simulink model "DroneControl_copy"  (R2023a)
settings: Solver=VariableStepAuto  StartTime=0.0  StopTime=Tfinal  RelTol=1e-3
values from neighbouring files (symbols this model uses):
  body_rate_0 = [0 0 ... (first row only)    [XYZsignal_copy.m]
  Euler_0 = [0 0 ... (first row only)    [XYZsignal_copy.m]
  g = [0;0;-9.8]    [XYZsignal_copy.m]
  I = [[0.1,0,0];[0,0.1,0];[0,0,0.08]]    [XYZsignal_copy.m]
  m = 0.2    [XYZsignal_copy.m]    (also in animation_copy.m = T_V1toI*T_V2toV1*T_BtoV2)
  surround_rate = 0    [XYZsignal_copy.m]
  ts = 0.01    [XYZsignal_copy.m]
  Xcmd1 = timeseries(sigX1(2:end,:),sigX1(1,:))    [XYZsignal_copy.m]
  Xcmd2 = timeseries(sigX2(2:end,:),sigX2(1,:))    [XYZsignal_copy.m]
  XYZ_0 = [0.1 10.1 ... (first row only)    [XYZsignal_copy.m]
  Ycmd1 = timeseries(sigY1(2:end,:),sigY1(1,:))    [XYZsignal_copy.m]
  Ycmd2 = timeseries(sigY2(2:end,:),sigY2(1,:))    [XYZsignal_copy.m]
libraries: slpidlib x36, vrlib x4, simulink_extras x2
(part 1 of 5)
settings Model: NumberOfSteps=10  Creator=blaze8871  LastModifiedBy=sujay
settings SolverCC: AlgebraicLoopSolver=TrustRegion
settings DataIOCC: SaveTime=off
settings DebuggingCC: UnconnectedInputMsg=warning  UnconnectedOutputMsg=warning  UnconnectedLineMsg=warning
settings ModelReferenceCC: EnableRefExpFcnMdlSchedulingChecks=on

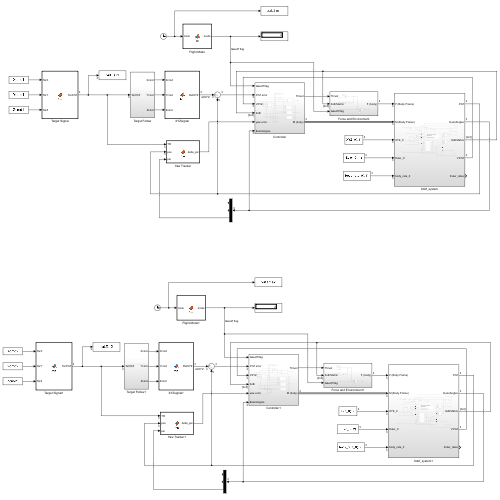
[thumbnail: Simulink's stored preview of the top-level diagram]
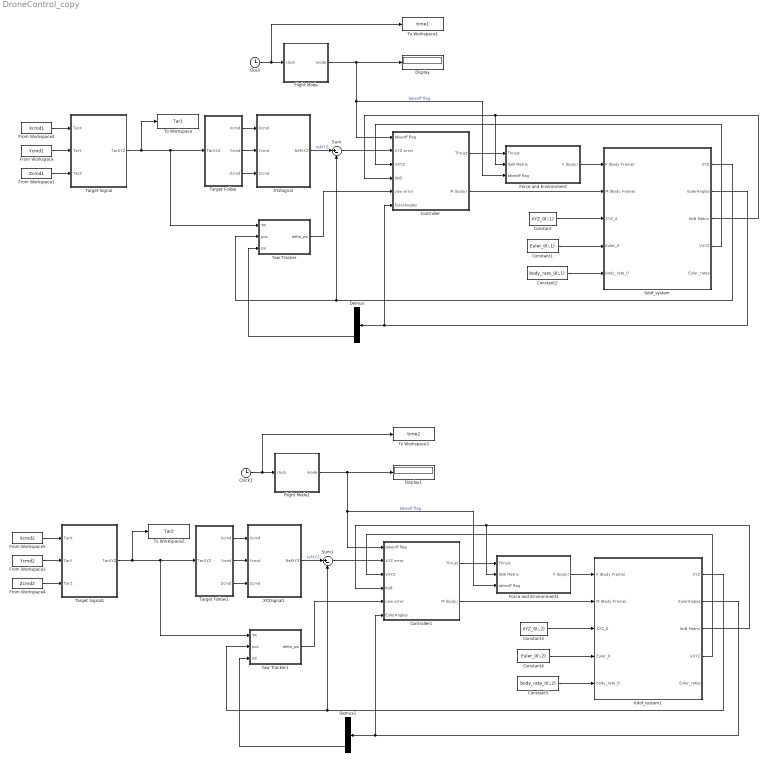
== system DroneControl_copy ==
  6dof_system : Subsystem
  6dof_system1 : Subsystem
  Clock : Clock
  Clock1 : Clock
  Constant : Constant  Value=XYZ_0(:,1)  SampleTime=0.01
  Constant1 : Constant  Value=Euler_0(:,1)  SampleTime=0.01
  Constant2 : Constant  Value=body_rate_0(:,1)  SampleTime=0.01
  Constant3 : Constant  Value=XYZ_0(:,2)  SampleTime=0.01
  Constant4 : Constant  Value=Euler_0(:,2)  SampleTime=0.01
  Constant5 : Constant  Value=body_rate_0(:,2)  SampleTime=0.01
  Controller : Subsystem
  Controller1 : Subsystem
  Demux : Demux  Outputs=3
  Demux1 : Demux  Outputs=3
  Display : Display
  Display1 : Display
  Flight Mode : MATLAB Function  TreatAsAtomicUnit=on
  Flight Mode1 : MATLAB Function  TreatAsAtomicUnit=on
  Force and Environment : Subsystem
  Force and Environment1 : Subsystem
  From Workspace : FromWorkspace  VariableName=Ycmd1  SampleTime=ts
  From Workspace1 : FromWorkspace  VariableName=Zcmd1  SampleTime=ts
  From Workspace2 : FromWorkspace  VariableName=Xcmd1  SampleTime=ts
  From Workspace3 : FromWorkspace  VariableName=Ycmd2  SampleTime=ts
  From Workspace4 : FromWorkspace  VariableName=Zcmd2  SampleTime=ts
  From Workspace5 : FromWorkspace  VariableName=Xcmd2  SampleTime=ts
  Sum : Sum  Inputs=|+-
  Sum1 : Sum  Inputs=|+-
  Target Follow : Subsystem
  Target Follow1 : Subsystem
  Target Signal : MATLAB Function  TreatAsAtomicUnit=on
  Target Signal1 : MATLAB Function  TreatAsAtomicUnit=on
  To Workspace : ToWorkspace  VariableName=Tar1  SampleTime=ts
  To Workspace1 : ToWorkspace  VariableName=time1  SampleTime=ts
  To Workspace2 : ToWorkspace  VariableName=Tar2  SampleTime=ts
  To Workspace3 : ToWorkspace  VariableName=time2  SampleTime=ts
  XYZsignal : MATLAB Function  TreatAsAtomicUnit=on
  XYZsignal1 : MATLAB Function  TreatAsAtomicUnit=on
  Yaw Tracker : MATLAB Function  TreatAsAtomicUnit=on
  Yaw Tracker1 : MATLAB Function  TreatAsAtomicUnit=on
  wires:
  Constant/1 -> 6dof_system/3(XYZ_0)
  Constant1/1 -> 6dof_system/4(Euler_0)
  Constant2/1 -> 6dof_system/5(body_rate_0)
  6dof_system/3(ItoB Matrix) -> Force and Environment/2(ItoB Matrix), Controller/4(ItoB)
  XYZsignal/1(RefXYZ) -> Sum/1  "refXYZ"
  6dof_system/1(XYZ) -> Sum/2, Yaw Tracker/2(pos)
  Clock/1 -> To Workspace1/1, Flight Mode/1(clock)
  Flight Mode/1(mode) -> Controller/1(takeoff flag), Force and Environment/3(takeoff flag), Display/1  "takeoff flag"
  Force and Environment/1(F (body)) -> 6dof_system/1(F (Body Frame))
  6dof_system/2(EulerAngles) -> Controller/6(EulerAngles), Demux/1
  Sum/1 -> Controller/2(XYZ error)
  6dof_system/4(VXYZ) -> Controller/3(VXYZ)
  Controller/2(M (body)) -> 6dof_system/2(M (Body Frame))
  Controller/1(Thrust) -> Force and Environment/1(Thrust)
  Demux/3 -> Yaw Tracker/3(psi)
  Yaw Tracker/1(delta_psi) -> Controller/5(yaw error)
  Target Signal/1(TarXYZ) -> To Workspace/1, Target Follow/1(TarXYZ), Yaw Tracker/1(TR)
  From Workspace2/1 -> Target Signal/1(TarX)
  From Workspace/1 -> Target Signal/2(TarY)
  From Workspace1/1 -> Target Signal/3(TarZ)
  Target Follow/1(Xcmd) -> XYZsignal/1(Xcmd)
  Target Follow/2(Ycmd) -> XYZsignal/2(Ycmd)
  Target Follow/3(Zcmd) -> XYZsignal/3(Zcmd)
  Controller1/2(M (body)) -> 6dof_system1/2(M (Body Frame))
  Demux1/3 -> Yaw Tracker1/3(psi)
  Yaw Tracker1/1(delta_psi) -> Controller1/5(yaw error)
  Controller1/1(Thrust) -> Force and Environment1/1(Thrust)
  From Workspace3/1 -> Target Signal1/2(TarY)
  Force and Environment1/1(F (body)) -> 6dof_system1/1(F (Body Frame))
  Target Signal1/1(TarXYZ) -> To Workspace2/1, Target Follow1/1(TarXYZ), Yaw Tracker1/1(TR)
  Target Follow1/3(Zcmd) -> XYZsignal1/3(Zcmd)
  Target Follow1/1(Xcmd) -> XYZsignal1/1(Xcmd)
  From Workspace4/1 -> Target Signal1/3(TarZ)
  From Workspace5/1 -> Target Signal1/1(TarX)
  Constant3/1 -> 6dof_system1/3(XYZ_0)
  6dof_system1/4(VXYZ) -> Controller1/3(VXYZ)
  6dof_system1/2(EulerAngles) -> Controller1/6(EulerAngles), Demux1/1
  XYZsignal1/1(RefXYZ) -> Sum1/1  "refXYZ"
  6dof_system1/3(ItoB Matrix) -> Force and Environment1/2(ItoB Matrix), Controller1/4(ItoB)
  Flight Mode1/1(mode) -> Controller1/1(takeoff flag), Force and Environment1/3(takeoff flag), Display1/1  "takeoff flag"
  Sum1/1 -> Controller1/2(XYZ error)
  Constant4/1 -> 6dof_system1/4(Euler_0)
  Constant5/1 -> 6dof_system1/5(body_rate_0)
  Clock1/1 -> To Workspace3/1, Flight Mode1/1(clock)
  Target Follow1/2(Ycmd) -> XYZsignal1/2(Ycmd)
  6dof_system1/1(XYZ) -> Sum1/2, Yaw Tracker1/2(pos)

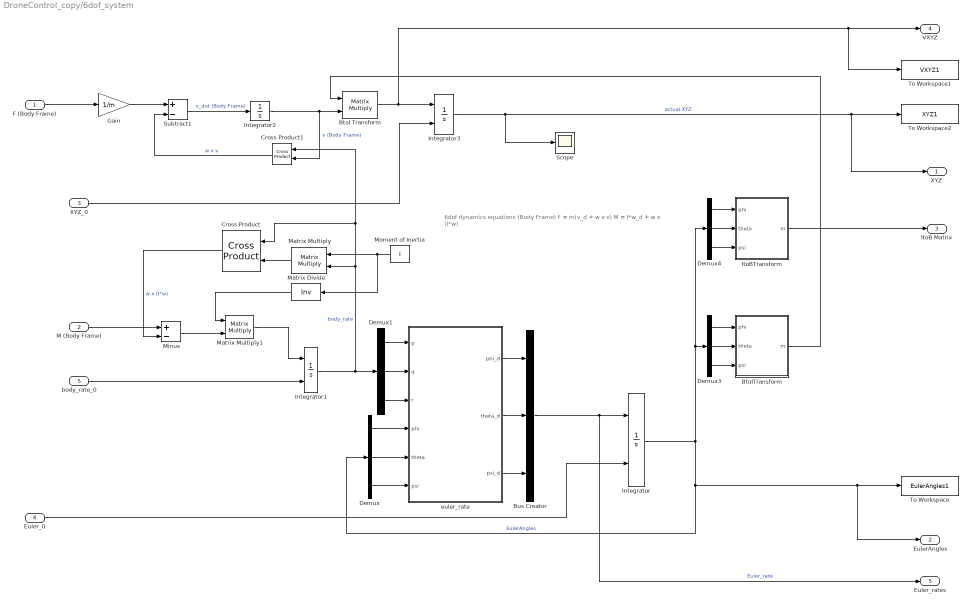
== system DroneControl_copy/6dof_system ==
  note: 6dof dynamics equations
      | (Body Frame)
      |
      | F = m(v_d + w x v)
      | M = I*w_d + w x (I*w)
  F (Body Frame) : Inport
  M (Body Frame) : Inport  Port=2
  XYZ_0 : Inport  Port=3
  Euler_0 : Inport  Port=4
  body_rate_0 : Inport  Port=5
  BtoI Transform : Product  Multiplication=Matrix(*)
  BtoITransform : MATLAB Function  TreatAsAtomicUnit=on
  Bus Creator : BusCreator  Inputs=3
  Cross Product : vrlib/Utilities/Cross Product
  Cross Product1 : vrlib/Utilities/Cross Product
  Demux{,1,3..4} (4 alike) : Demux  Outputs=3
  Gain : Gain  Gain=1/m
  Integrator : Integrator  InitialConditionSource=external  ContinuousStateAttributes='EulerAngle'
  Integrator1 : Integrator  InitialConditionSource=external  ContinuousStateAttributes='EulerAngle'
  Integrator2 : Integrator
  Integrator3 : Integrator  InitialConditionSource=external
  ItoBTransform : MATLAB Function  TreatAsAtomicUnit=on
  Matrix Divide : Product  Inputs=/  Multiplication=Matrix(*)
  Matrix Multiply : Product  Multiplication=Matrix(*)
  Matrix Multiply1 : Product  Multiplication=Matrix(*)
  Minus : Sum  Inputs=+-
  Moment of Inertia : Constant  Value=I
  Scope : Scope
  Subtract1 : Sum  Inputs=+-
  To Workspace : ToWorkspace  VariableName=EulerAngles1  SampleTime=ts
  To Workspace1 : ToWorkspace  VariableName=VXYZ1  SampleTime=ts
  To Workspace2 : ToWorkspace  VariableName=XYZ1  SampleTime=ts
  euler_rate : MATLAB Function  TreatAsAtomicUnit=on
  XYZ : Outport
  EulerAngles : Outport  Port=2
  ItoB Matrix : Outport  Port=3
  VXYZ : Outport  Port=4
  Euler_rates : Outport  Port=5
  wires:
  F (Body Frame)/1 -> Gain/1
  Demux4/2 -> ItoBTransform/2(theta)
  euler_rate/1(phi_d) -> Bus Creator/1
  BtoITransform/1(m) -> BtoI Transform/1
  Bus Creator/1 -> Euler_rates/1, Integrator/1  "Euler_rate"
  Matrix Multiply/1 -> Cross Product/2
  Moment of Inertia/1 -> Matrix Divide/1, Matrix Multiply/1
  Demux3/2 -> BtoITransform/2(theta)
  Demux/2 -> euler_rate/5(theta)
  Demux4/1 -> ItoBTransform/1(phi)
  Subtract1/1 -> Integrator2/1  "v_dot (Body Frame)"
  Cross Product1/1 -> Subtract1/2  "w x v"
  Demux1/1 -> euler_rate/1(p)
  Demux/3 -> euler_rate/6(psi)
  euler_rate/2(theta_d) -> Bus Creator/2
  Euler_0/1 -> Integrator/2
  Integrator3/1 -> XYZ/1, To Workspace2/1, Scope/1  "actual XYZ"
  Cross Product/1 -> Minus/2  "w x (I*w)"
  M (Body Frame)/1 -> Minus/1
  body_rate_0/1 -> Integrator1/2
  Demux3/3 -> BtoITransform/3(psi)
  euler_rate/3(psi_d) -> Bus Creator/3
  Demux4/3 -> ItoBTransform/3(psi)
  Gain/1 -> Subtract1/1
  Demux3/1 -> BtoITransform/1(phi)
  Demux1/3 -> euler_rate/3(r)
  XYZ_0/1 -> Integrator3/2
  Integrator/1 -> EulerAngles/1, To Workspace/1, Demux/1, Demux4/1, Demux3/1  "EulerAngles"
  Demux/1 -> euler_rate/4(phi)
  Integrator2/1 -> BtoI Transform/2, Cross Product1/2  "v (Body Frame)"
  Integrator1/1 -> Cross Product1/1, Cross Product/1, Matrix Multiply/2, Demux1/1  "body_rate"
  Demux1/2 -> euler_rate/2(q)
  ItoBTransform/1(m) -> ItoB Matrix/1
  BtoI Transform/1 -> To Workspace1/1, VXYZ/1, Integrator3/1
  Minus/1 -> Matrix Multiply1/2
  Matrix Multiply1/1 -> Integrator1/1
  Matrix Divide/1 -> Matrix Multiply1/1

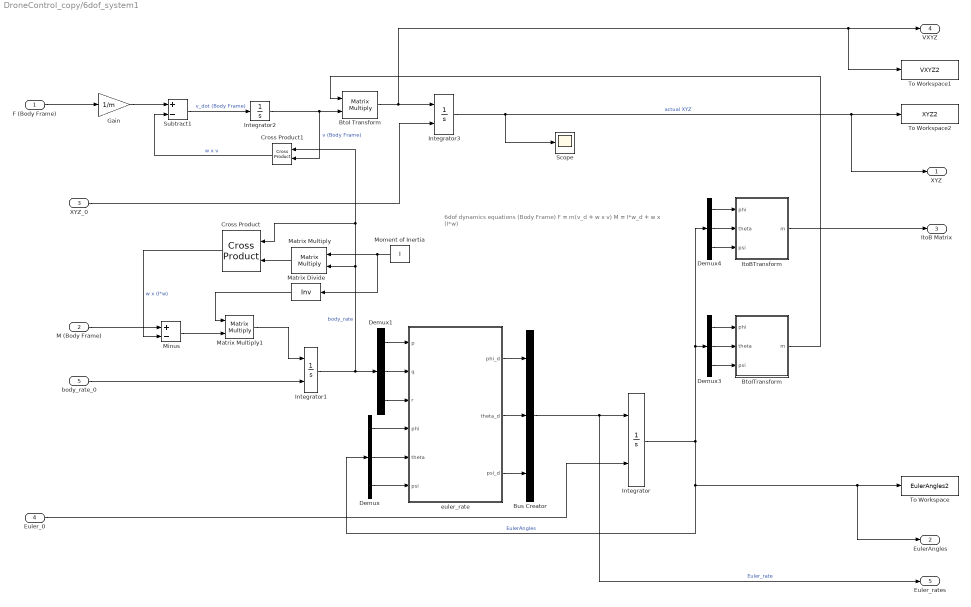
== system DroneControl_copy/6dof_system1 ==
  note: 6dof dynamics equations
      | (Body Frame)
      |
      | F = m(v_d + w x v)
      | M = I*w_d + w x (I*w)
  F (Body Frame) : Inport
  M (Body Frame) : Inport  Port=2
  XYZ_0 : Inport  Port=3
  Euler_0 : Inport  Port=4
  body_rate_0 : Inport  Port=5
  BtoI Transform : Product  Multiplication=Matrix(*)
  BtoITransform : MATLAB Function  TreatAsAtomicUnit=on
  Bus Creator : BusCreator  Inputs=3
  Cross Product : vrlib/Utilities/Cross Product
  Cross Product1 : vrlib/Utilities/Cross Product
  Demux{,1,3..4} (4 alike) : Demux  Outputs=3
  Gain : Gain  Gain=1/m
  Integrator : Integrator  InitialConditionSource=external  ContinuousStateAttributes='EulerAngle'
  Integrator1 : Integrator  InitialConditionSource=external  ContinuousStateAttributes='EulerAngle'
  Integrator2 : Integrator
  Integrator3 : Integrator  InitialConditionSource=external
  ItoBTransform : MATLAB Function  TreatAsAtomicUnit=on
  Matrix Divide : Product  Inputs=/  Multiplication=Matrix(*)
  Matrix Multiply : Product  Multiplication=Matrix(*)
  Matrix Multiply1 : Product  Multiplication=Matrix(*)
  Minus : Sum  Inputs=+-
  Moment of Inertia : Constant  Value=I
  Scope : Scope
  Subtract1 : Sum  Inputs=+-
  To Workspace : ToWorkspace  VariableName=EulerAngles2  SampleTime=ts
  To Workspace1 : ToWorkspace  VariableName=VXYZ2  SampleTime=ts
  To Workspace2 : ToWorkspace  VariableName=XYZ2  SampleTime=ts
  euler_rate : MATLAB Function  TreatAsAtomicUnit=on
  XYZ : Outport
  EulerAngles : Outport  Port=2
  ItoB Matrix : Outport  Port=3
  VXYZ : Outport  Port=4
  Euler_rates : Outport  Port=5
  wires:
  F (Body Frame)/1 -> Gain/1
  Demux4/2 -> ItoBTransform/2(theta)
  euler_rate/1(phi_d) -> Bus Creator/1
  BtoITransform/1(m) -> BtoI Transform/1
  Bus Creator/1 -> Euler_rates/1, Integrator/1  "Euler_rate"
  Matrix Multiply/1 -> Cross Product/2
  Moment of Inertia/1 -> Matrix Divide/1, Matrix Multiply/1
  Demux3/2 -> BtoITransform/2(theta)
  Demux/2 -> euler_rate/5(theta)
  Demux4/1 -> ItoBTransform/1(phi)
  Subtract1/1 -> Integrator2/1  "v_dot (Body Frame)"
  Cross Product1/1 -> Subtract1/2  "w x v"
  Demux1/1 -> euler_rate/1(p)
  Demux/3 -> euler_rate/6(psi)
  euler_rate/2(theta_d) -> Bus Creator/2
  Euler_0/1 -> Integrator/2
  Integrator3/1 -> XYZ/1, To Workspace2/1, Scope/1  "actual XYZ"
  Cross Product/1 -> Minus/2  "w x (I*w)"
  M (Body Frame)/1 -> Minus/1
  body_rate_0/1 -> Integrator1/2
  Demux3/3 -> BtoITransform/3(psi)
  euler_rate/3(psi_d) -> Bus Creator/3
  Demux4/3 -> ItoBTransform/3(psi)
  Gain/1 -> Subtract1/1
  Demux3/1 -> BtoITransform/1(phi)
  Demux1/3 -> euler_rate/3(r)
  XYZ_0/1 -> Integrator3/2
  Integrator/1 -> EulerAngles/1, To Workspace/1, Demux/1, Demux4/1, Demux3/1  "EulerAngles"
  Demux/1 -> euler_rate/4(phi)
  Integrator2/1 -> BtoI Transform/2, Cross Product1/2  "v (Body Frame)"
  Integrator1/1 -> Cross Product1/1, Cross Product/1, Matrix Multiply/2, Demux1/1  "body_rate"
  Demux1/2 -> euler_rate/2(q)
  ItoBTransform/1(m) -> ItoB Matrix/1
  BtoI Transform/1 -> To Workspace1/1, VXYZ/1, Integrator3/1
  Minus/1 -> Matrix Multiply1/2
  Matrix Multiply1/1 -> Integrator1/1
  Matrix Divide/1 -> Matrix Multiply1/1

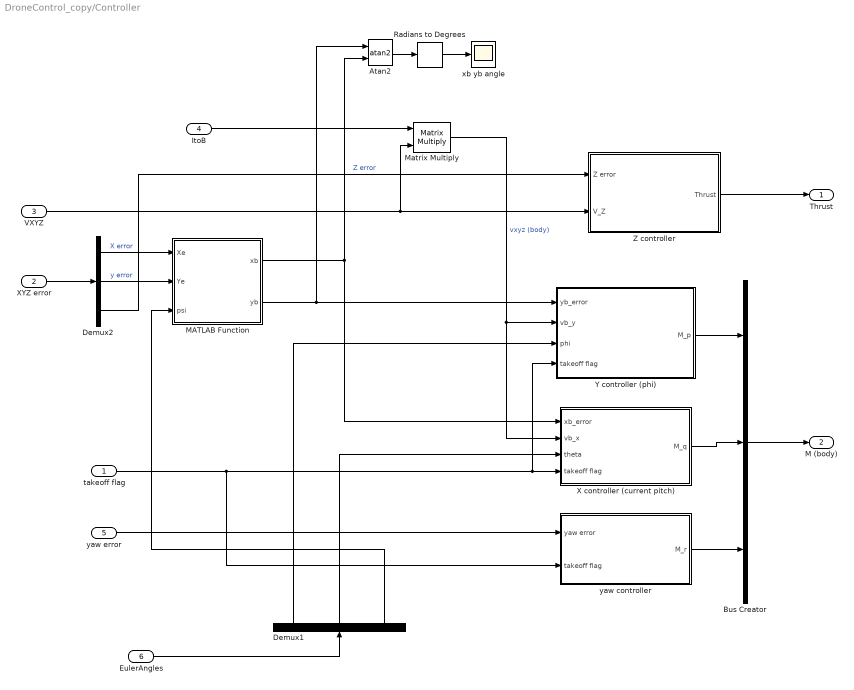
== system DroneControl_copy/Controller ==
  takeoff flag : Inport
  XYZ error : Inport  Port=2
  VXYZ : Inport  Port=3
  ItoB : Inport  Port=4
  yaw error : Inport  Port=5
  EulerAngles : Inport  Port=6
  Atan2 : Trigonometry  Operator=atan2
  Bus Creator : BusCreator  Inputs=3
  Demux1 : Demux  Outputs=3
  Demux2 : Demux  Outputs=3
  MATLAB Function : MATLAB Function  TreatAsAtomicUnit=on
  Matrix Multiply : Product  Multiplication=Matrix(*)
  Radians to Degrees : simulink_extras/Transformations/Radians to Degrees
  X controller (current pitch) : Subsystem
  Y controller (phi) : Subsystem
  Z controller : Subsystem
  xb yb angle : Scope
  "yaw controller " : Subsystem
  Thrust : Outport
  M (body) : Outport  Port=2
  wires:
  Bus Creator/1 -> M (body)/1
  VXYZ/1 -> Z controller/2(V_Z), Matrix Multiply/2
  "yaw controller "/1(M_r) -> Bus Creator/3
  XYZ error/1 -> Demux2/1
  Demux1/1 -> Y controller (phi)/3(phi)
  Demux1/2 -> X controller (current pitch)/3(theta)
  Demux2/3 -> Z controller/1(Z error)  "Z error"
  takeoff flag/1 -> Y controller (phi)/4(takeoff flag), X controller (current pitch)/4(takeoff flag), "yaw controller "/2(takeoff flag)
  EulerAngles/1 -> Demux1/1
  Y controller (phi)/1(M_p) -> Bus Creator/1
  Demux1/3 -> MATLAB Function/3(psi)
  Z controller/1(Thrust) -> Thrust/1
  Demux2/2 -> MATLAB Function/2(Ye)  "y error"
  yaw error/1 -> "yaw controller "/1(yaw error)
  Demux2/1 -> MATLAB Function/1(Xe)  "X error"
  X controller (current pitch)/1(M_q) -> Bus Creator/2
  MATLAB Function/1(xb) -> X controller (current pitch)/1("xb_error "), Atan2/2
  MATLAB Function/2(yb) -> Atan2/1, Y controller (phi)/1("yb_error ")
  Atan2/1 -> Radians to Degrees/1
  Radians to Degrees/1 -> xb yb angle/1
  ItoB/1 -> Matrix Multiply/1
  Matrix Multiply/1 -> X controller (current pitch)/2(vb_x), Y controller (phi)/2(vb_y)  "vxyz (body)"

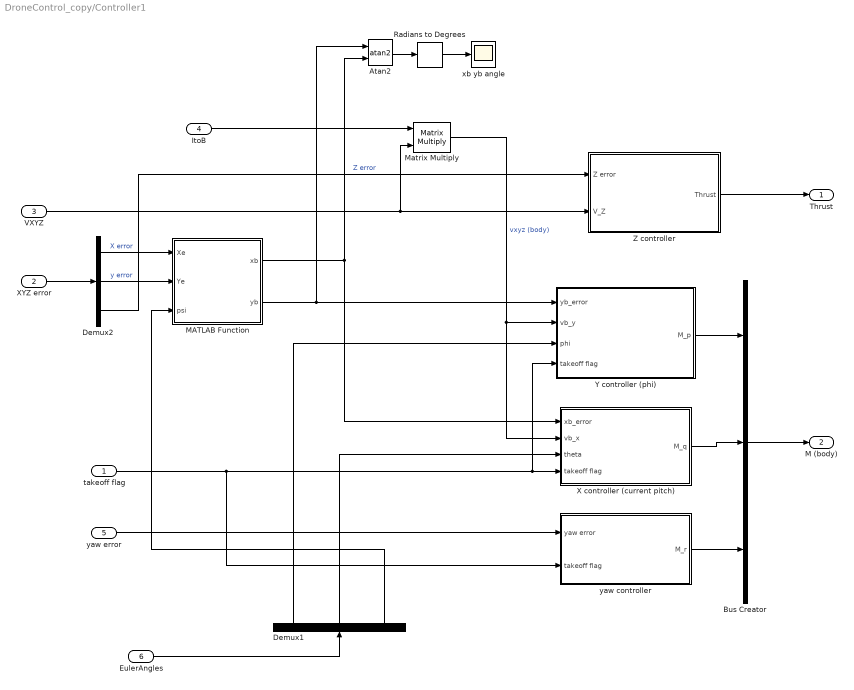
== system DroneControl_copy/Controller1 ==
  takeoff flag : Inport
  XYZ error : Inport  Port=2
  VXYZ : Inport  Port=3
  ItoB : Inport  Port=4
  yaw error : Inport  Port=5
  EulerAngles : Inport  Port=6
  Atan2 : Trigonometry  Operator=atan2
  Bus Creator : BusCreator  Inputs=3
  Demux1 : Demux  Outputs=3
  Demux2 : Demux  Outputs=3
  MATLAB Function : MATLAB Function  TreatAsAtomicUnit=on
  Matrix Multiply : Product  Multiplication=Matrix(*)
  Radians to Degrees : simulink_extras/Transformations/Radians to Degrees
  X controller (current pitch) : Subsystem
  Y controller (phi) : Subsystem
  Z controller : Subsystem
  xb yb angle : Scope
  "yaw controller " : Subsystem
  Thrust : Outport
  M (body) : Outport  Port=2
  wires:
  Bus Creator/1 -> M (body)/1
  VXYZ/1 -> Z controller/2(V_Z), Matrix Multiply/2
  "yaw controller "/1(M_r) -> Bus Creator/3
  XYZ error/1 -> Demux2/1
  Demux1/1 -> Y controller (phi)/3(phi)
  Demux1/2 -> X controller (current pitch)/3(theta)
  Demux2/3 -> Z controller/1(Z error)  "Z error"
  takeoff flag/1 -> Y controller (phi)/4(takeoff flag), X controller (current pitch)/4(takeoff flag), "yaw controller "/2(takeoff flag)
  EulerAngles/1 -> Demux1/1
  Y controller (phi)/1(M_p) -> Bus Creator/1
  Demux1/3 -> MATLAB Function/3(psi)
  Z controller/1(Thrust) -> Thrust/1
  Demux2/2 -> MATLAB Function/2(Ye)  "y error"
  yaw error/1 -> "yaw controller "/1(yaw error)
  Demux2/1 -> MATLAB Function/1(Xe)  "X error"
  X controller (current pitch)/1(M_q) -> Bus Creator/2
  MATLAB Function/1(xb) -> X controller (current pitch)/1("xb_error "), Atan2/2
  MATLAB Function/2(yb) -> Atan2/1, Y controller (phi)/1("yb_error ")
  Atan2/1 -> Radians to Degrees/1
  Radians to Degrees/1 -> xb yb angle/1
  ItoB/1 -> Matrix Multiply/1
  Matrix Multiply/1 -> X controller (current pitch)/2(vb_x), Y controller (phi)/2(vb_y)  "vxyz (body)"

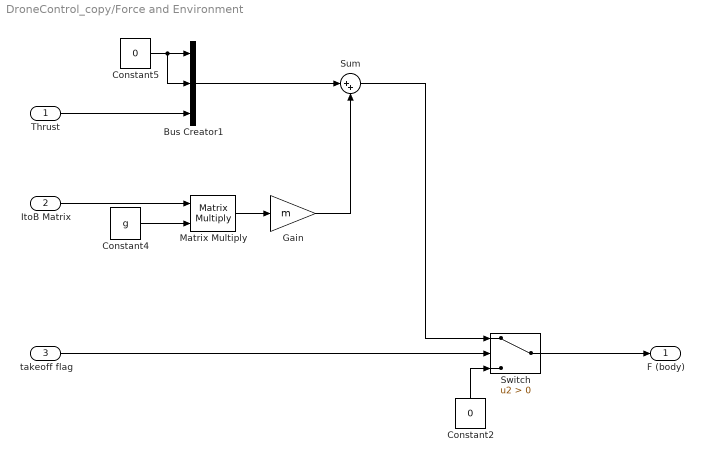
== system DroneControl_copy/Force and Environment ==
  Thrust : Inport
  ItoB Matrix : Inport  Port=2
  takeoff flag : Inport  Port=3
  Bus Creator1 : BusCreator  Inputs=3
  Constant2 : Constant  Value=0  SampleTime=0.01
  Constant4 : Constant  Value=g  SampleTime=0.01
  Constant5 : Constant  Value=0  SampleTime=0.01
  Gain : Gain  Gain=m
  Matrix Multiply : Product  Multiplication=Matrix(*)
  Sum : Sum  Inputs=|++
  Switch : Switch  Criteria=u2 > Threshold  SaturateOnIntegerOverflow=off  InputSameDT=off
  F (body) : Outport
  wires:
  Thrust/1 -> Bus Creator1/3
  Bus Creator1/1 -> Sum/1
  Constant4/1 -> Matrix Multiply/2
  ItoB Matrix/1 -> Matrix Multiply/1
  Constant5/1 -> Bus Creator1/2, Bus Creator1/1
  takeoff flag/1 -> Switch/2
  Constant2/1 -> Switch/3
  Matrix Multiply/1 -> Gain/1
  Sum/1 -> Switch/1
  Switch/1 -> F (body)/1
  Gain/1 -> Sum/2

== system DroneControl_copy/Force and Environment1 ==
  Thrust : Inport
  ItoB Matrix : Inport  Port=2
  takeoff flag : Inport  Port=3
  Bus Creator1 : BusCreator  Inputs=3
  Constant2 : Constant  Value=0  SampleTime=0.01
  Constant4 : Constant  Value=g  SampleTime=0.01
  Constant5 : Constant  Value=0  SampleTime=0.01
  Gain : Gain  Gain=m
  Matrix Multiply : Product  Multiplication=Matrix(*)
  Sum : Sum  Inputs=|++
  Switch : Switch  Criteria=u2 > Threshold  SaturateOnIntegerOverflow=off  InputSameDT=off
  F (body) : Outport
  wires:
  Thrust/1 -> Bus Creator1/3
  Bus Creator1/1 -> Sum/1
  Constant4/1 -> Matrix Multiply/2
  ItoB Matrix/1 -> Matrix Multiply/1
  Constant5/1 -> Bus Creator1/2, Bus Creator1/1
  takeoff flag/1 -> Switch/2
  Constant2/1 -> Switch/3
  Matrix Multiply/1 -> Gain/1
  Sum/1 -> Switch/1
  Switch/1 -> F (body)/1
  Gain/1 -> Sum/2

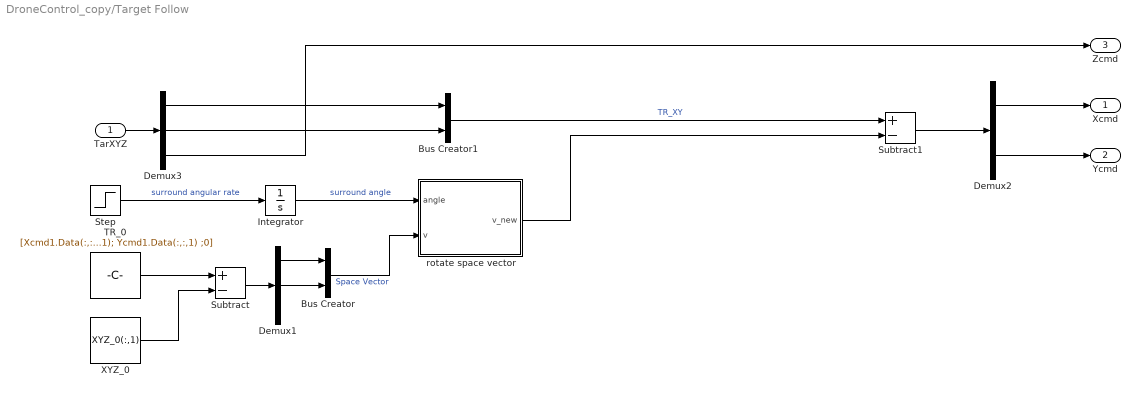
== system DroneControl_copy/Target Follow ==
  TarXYZ : Inport
  Bus Creator : BusCreator  Inputs=2
  Bus Creator1 : BusCreator  Inputs=2
  Demux1 : Demux  Outputs=3
  Demux2 : Demux  Outputs=2
  Demux3 : Demux  Outputs=3
  Integrator : Integrator
  Step : Step  Time=2  After=surround_rate  SampleTime=0
  Subtract : Sum  Inputs=+-
  Subtract1 : Sum  Inputs=+-
  TR_0 : Constant  Value=[Xcmd1.Data(:,:,1); Ycmd1.Data(:,:,1) ;0]
  XYZ_0 : Constant  Value=XYZ_0(:,1)
  rotate space vector : MATLAB Function  TreatAsAtomicUnit=on
  Xcmd : Outport
  Ycmd : Outport  Port=2
  Zcmd : Outport  Port=3
  wires:
  Subtract1/1 -> Demux2/1
  Demux2/2 -> Ycmd/1
  TR_0/1 -> Subtract/1
  Demux1/2 -> Bus Creator/2
  Bus Creator1/1 -> Subtract1/1  "TR_XY"
  TarXYZ/1 -> Demux3/1
  Demux3/2 -> Bus Creator1/2
  Subtract/1 -> Demux1/1
  Demux3/3 -> Zcmd/1
  Demux2/1 -> Xcmd/1
  Demux1/1 -> Bus Creator/1
  Demux3/1 -> Bus Creator1/1
  Bus Creator/1 -> rotate space vector/2(v)  "Space Vector"
  XYZ_0/1 -> Subtract/2
  Step/1 -> Integrator/1  "surround angular rate"
  Integrator/1 -> rotate space vector/1(angle)  "surround angle"
  rotate space vector/1(v_new) -> Subtract1/2

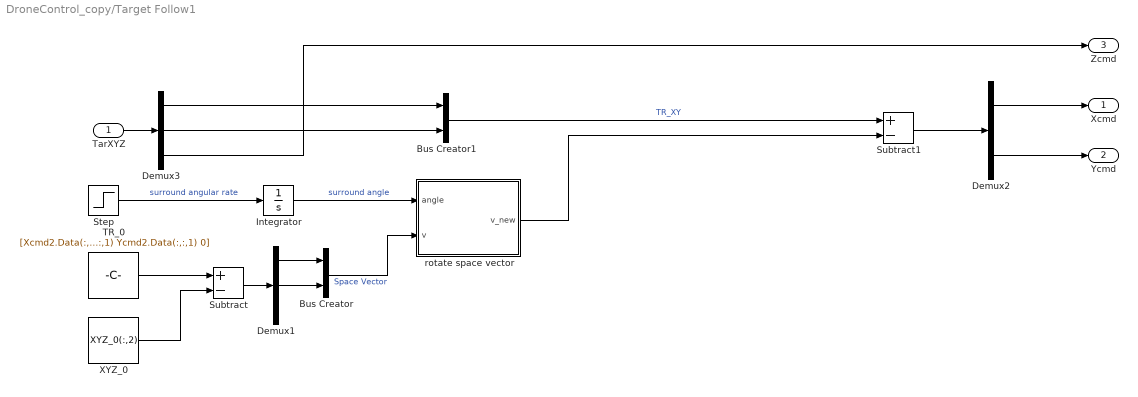
== system DroneControl_copy/Target Follow1 ==
  TarXYZ : Inport
  Bus Creator : BusCreator  Inputs=2
  Bus Creator1 : BusCreator  Inputs=2
  Demux1 : Demux  Outputs=3
  Demux2 : Demux  Outputs=2
  Demux3 : Demux  Outputs=3
  Integrator : Integrator
  Step : Step  Time=2  After=surround_rate  SampleTime=0
  Subtract : Sum  Inputs=+-
  Subtract1 : Sum  Inputs=+-
  TR_0 : Constant  Value=[Xcmd2.Data(:,:,1) Ycmd2.Data(:,:,1) 0]
  XYZ_0 : Constant  Value=XYZ_0(:,2)
  rotate space vector : MATLAB Function  TreatAsAtomicUnit=on
  Xcmd : Outport
  Ycmd : Outport  Port=2
  Zcmd : Outport  Port=3
  wires:
  Subtract1/1 -> Demux2/1
  Demux2/2 -> Ycmd/1
  TR_0/1 -> Subtract/1
  Demux1/2 -> Bus Creator/2
  Bus Creator1/1 -> Subtract1/1  "TR_XY"
  TarXYZ/1 -> Demux3/1
  Demux3/2 -> Bus Creator1/2
  Subtract/1 -> Demux1/1
  Demux3/3 -> Zcmd/1
  Demux2/1 -> Xcmd/1
  Demux1/1 -> Bus Creator/1
  Demux3/1 -> Bus Creator1/1
  Bus Creator/1 -> rotate space vector/2(v)  "Space Vector"
  XYZ_0/1 -> Subtract/2
  Step/1 -> Integrator/1  "surround angular rate"
  Integrator/1 -> rotate space vector/1(angle)  "surround angle"
  rotate space vector/1(v_new) -> Subtract1/2
